simulink model "HystressisCurrentController"  (R2023a)
settings: Solver=VariableStepAuto  StartTime=0.0  StopTime=2  MaxStep=.001  RelTol=1e-3
values from neighbouring files (symbols this model uses):
  B = .005752    (= 0.005752)    [parameters.m]
  Delta = 0.1    [parameters.m]
  J = .02    (= 0.02)    [parameters.m]
  lambda_r_rated = (Vph_rms/(2*pi*Freq))*(1-sigma)    [parameters.m]
  Llr = .005974    (= 0.005974)    [parameters.m]
  Lls = .005974    (= 0.005974)    [parameters.m]
  Lm = .2037    (= 0.2037)    [parameters.m]
  Lr = Lm+Llr    (= 0.209674)    [parameters.m]
  P = 4    [parameters.m]
  Rs = 1.115    [parameters.m]
  Tr = Lr/Rr    (= 0.193604801477)    [parameters.m]
  Vdc = 400    [parameters.m]
libraries: spsMosfetLib x6, spsabctoAlphaBetaZeroLib x4, slpidlib x4, spsAsynchronousMachineSIUnitsLib x1, spsDCVoltageSourceLib x1, spsGroundLib x1, SignalEditorBlockLib x1, spsThreePhaseVIMeasurementLib x1, spsabctodq0Lib x1, sps_lib x1
settings Model: Creator=User  LastModifiedBy=User

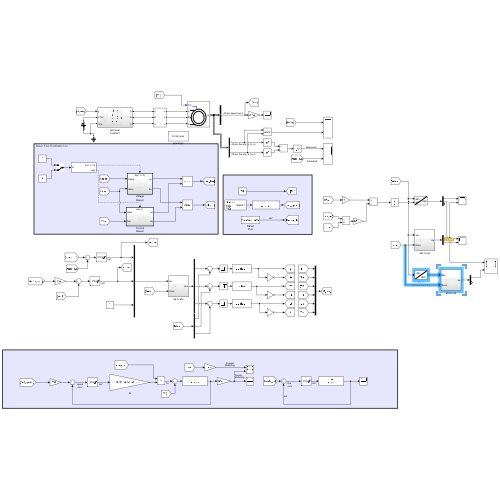
[thumbnail: Simulink's stored preview of the top-level diagram]
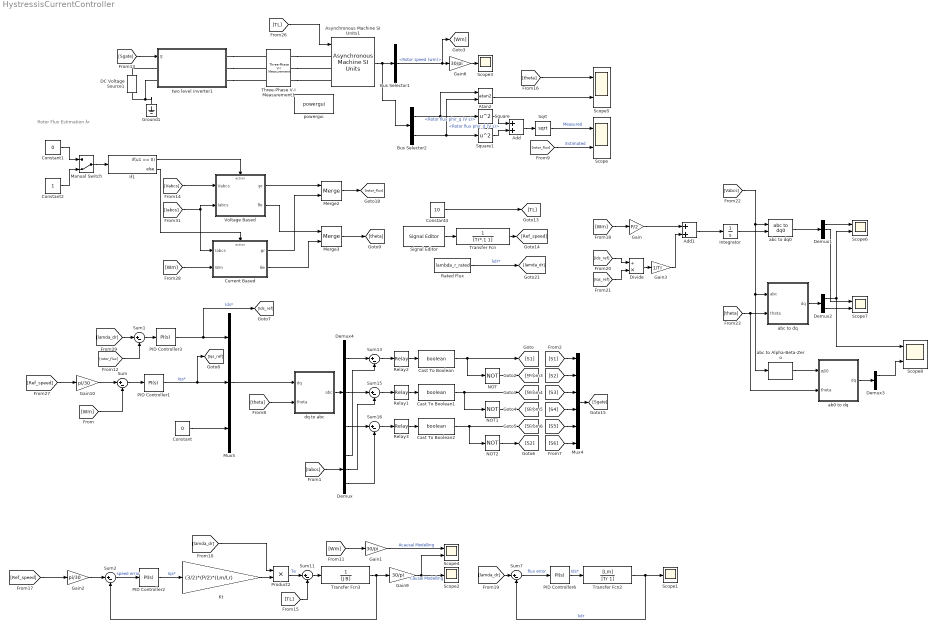
== system HystressisCurrentController ==
  note: Rotor Flux Estimation λr
  Add : Sum
  Add1 : Sum
  Asynchronous Machine SI Units1 : spsAsynchronousMachineSIUnitsLib/Asynchronous Machine SI Units  RotorType=Squirrel-cage  PresetModel="01:  5 HP   460 V 60Hz 1750 RPM"  MechanicalLoad=Torque Tm  ShowDetailedParameters=on  ReferenceFrame=Stationary  Units=SI  MeasurementBus=off  NominalParameters=[3730 460 60]  VoltageRatio=1  Stator=[1.115 0.005974]  Rotor=[1.083 0.005974]  Cage1=[0.4155 0.002066]  Cage2=[0.4168 0.0003495]  Lm=0.2037  Mechanical=[0.02 0.005752 2]  PolePairs=2  InitialConditions=[1 0 0 0 0 0 0 0]  SimulateSaturation=off  Saturation=[14.03593122, 27.81365428, 53.79336849, 72.68890987, 97.98006896, 148.6815601, 215.7428561, 302.9841135, 428.7778367 ; 230, 322, 414, 460, 506, 552, 598, 644, 690]  LoadFlowParameters=1492000  TsPowergui=0  TsBlock=-1  IterativeModel=Trapezoidal non iterative  IterativeDiscreteModel=Trapezoidal non iterative  Pmec=1.492e+006
  Atan2 : Trigonometry  Operator=atan2
  Bus Selector1 : BusSelector  OutputSignals=Mechanical.Rotor speed (wm)
  Bus Selector2 : BusSelector  OutputSignals=Rotor measurements.Rotor flux phir_q (V s),Rotor measurements.Rotor flux phir_d (V s)
  Cast To Boolean : DataTypeConversion  OutDataTypeStr=boolean  SaturateOnIntegerOverflow=off  RndMeth=Floor
  Cast To Boolean1 : DataTypeConversion  OutDataTypeStr=boolean  SaturateOnIntegerOverflow=off  RndMeth=Floor
  Cast To Boolean2 : DataTypeConversion  OutDataTypeStr=boolean  SaturateOnIntegerOverflow=off  RndMeth=Floor
  Constant : Constant  Value=0
  Constant1 : Constant  Value=0
  Constant2 : Constant
  Constant4 : Constant  Value=10
  Current Based : Subsystem
  DC Voltage Source1 : spsDCVoltageSourceLib/DC Voltage Source  Amplitude=Vdc  Measurements=None
  Demux : Demux  Outputs=3
  Demux1 : Demux  Outputs=3
  Demux2 : Demux  Outputs=2
  Demux3 : Demux  Outputs=2
  Demux4 : Demux  Outputs=3
  Divide : Product  Inputs=/*
  Gain : Gain  Gain=P/2
  Gain1 : Gain  Gain=30/pi
  Gain10 : Gain  Gain=pi/30
  Gain2 : Gain  Gain=pi/30
  Gain3 : Gain  Gain=1/Tr
  Gain6 : Gain  Gain=30/pi
  Gain9 : Gain  Gain=30/pi
  Ground1 : spsGroundLib/Ground  LConnTagsString=a
  If1 : If  IfExpression=u1 == 0
  Integrator : Integrator
  Kt : Gain  Gain=(3/2)*(P/2)*(Lm/Lr)
  Manual Switch : ManualSwitch  CurrentSetting=0
  Merge2 : Merge
  Merge3 : Merge
  Mux4 : Mux  Inputs=6
  Mux5 : Mux  Inputs=3
  NOT : Logic  Operator=NOT  IconShape=distinctive  AllPortsSameDT=off  OutDataTypeStr=boolean
  NOT1 : Logic  Operator=NOT  IconShape=distinctive  AllPortsSameDT=off  OutDataTypeStr=boolean
  NOT2 : Logic  Operator=NOT  IconShape=distinctive  AllPortsSameDT=off  OutDataTypeStr=boolean
  PID Controller1 : slpidlib/PID Controller  Controller=PI  Form=Parallel  TimeDomain=Continuous-time  UseExternalTs=off  SampleTime=-1  IntegratorMethod=Forward Euler  FilterMethod=Forward Euler  ControllerParametersSource=internal  P=5.28558902613874  I=47.3840704653277  UseKiTs=off  D=0  N=100  UseFilter=on  TunerSelectOption=Transfer Function Based (PID Tuner App)  InitialConditionSource=internal  InitialConditionForIntegrator=0  InitialConditionForFilter=0  DifferentiatorICPrevScaledInput=0  ExternalReset=none  TrackingMode=off  Kt=1  LimitOutput=on  SatLimitsSource=internal  UpperSaturationLimit=inf  LowerSaturationLimit=-inf  LinearizeAsGain=on  AntiWindupMode=clamping  Kb=1  LimitIntegrator=off  UpperIntegratorSaturationLimit=inf  LowerIntegratorSaturationLimit=-inf  POutMin=[]  POutMax=[]  IOutMin=[]  IOutMax=[]  DOutMin=[]  DOutMax=[]  NOutMin=[]  NOutMax=[]  SumOutMin=[]  SumOutMax=[]  SaturationOutMin=[]  SaturationOutMax=[]  PParamMin=[]  PParamMax=[]  IParamMin=[]  IParamMax=[]  DParamMin=[]  DParamMax=[]  NParamMin=[]  NParamMax=[]  KbParamMin=[]  KbParamMax=[]  KtParamMin=[]  KtParamMax=[]  KbOutMin=[]  KbOutMax=[]  KtOutMin=[]  KtOutMax=[]  IntegratorOutMin=[]  IntegratorOutMax=[]  FilterOutMin=[]  FilterOutMax=[]  SumI1OutMin=[]  SumI1OutMax=[]  SumI2OutMin=[]  SumI2OutMax=[]  SumI3OutMin=[]  SumI3OutMax=[]  SumI4OutMin=[]  SumI4OutMax=[]  SumDOutMin=[]  SumDOutMax=[]  DifferentiatorOutMin=[]  DifferentiatorOutMax=[]  FilterDiffOutCoefMin=[]  FilterDiffOutCoefMax=[]  ReciprocalOutMin=[]  ReciprocalOutMax=[]  SumDenOutMin=[]  SumDenOutMax=[]  SumNumOutMin=[]  SumNumOutMax=[]  DivideOutMin=[]  DivideOutMax=[]  UdiffTsProdOutMin=[]  UdiffTsProdOutMax=[]  NTsProdOutMin=[]  NTsProdOutMax=[]  UintegralTsProdOutMin=[]  UintegralTsProdOutMax=[]  UngainTsProdOutMin=[]  UngainTsProdOutMax=[]  ClampingZeroOutDataTypeStr=Inherit: Inherit via back propagation  ClampingZeroOutMin=[]  ClampingZeroOutMax=[]  FilterDenConstantOutDataTypeStr=Inherit: Inherit via back propagation  FilterDenConstantOutMin=[]  FilterDenConstantOutMax=[]  PCopyOutDataTypeStr=Inherit: Inherit via back propagation  PCopyOutMin=[]  PCopyOutMax=[]  NCopyOutDataTypeStr=Inherit: Inherit via back propagation  NCopyOutMin=[]  NCopyOutMax=[]  IntegratorContinuousStateAttributes=''  IntegratorStateMustResolveToSignalObject=off  IntegratorRTWStateStorageClass=Auto  FilterContinuousStateAttributes=''  FilterStateMustResolveToSignalObject=off  FilterRTWStateStorageClass=Auto  ParallelPVariant=InternalParameters  IdealPVariant=Disabled  IVariant=InternalParameters  DVariant=Disabled  IntegratorVariant=Continuous  SatVariant=Enabled  AWVariant=ContClampingParallel  PCopyVariant=Disabled  TRVariant=Disabled  FdbkBlocksVariant=Forward  IdealPFdbkVariant=Disabled  SatFdbkVariant=Disabled  DerivativeFilterVariant=Disabled  NVariant=Disabled  NCopyVariant=Disabled_SignalSpec  FilterICVariant=Disabled  IntegratorICVariant=InternalICs  ExternalResetVariant=Disabled  TRSumVariant=Passthrough  SumFdbkVariant=Disabled  SumVariant=Sum_PI  TsampFilterVariant=InternalTs  TsampNgainVariant=Passthrough  TsampIntegralVariant=Disabled_SignalSpec  ExternalSaturationOutDataTypeStr=Inherit: Same as second input
  PID Controller2 : slpidlib/PID Controller  Controller=PI  Form=Parallel  TimeDomain=Continuous-time  UseExternalTs=off  SampleTime=-1  IntegratorMethod=Forward Euler  FilterMethod=Forward Euler  ControllerParametersSource=internal  P=5.28558902613874  I=47.3840704653277  UseKiTs=off  D=0  N=100  UseFilter=on  TunerSelectOption=Transfer Function Based (PID Tuner App)  InitialConditionSource=internal  InitialConditionForIntegrator=0  InitialConditionForFilter=0  DifferentiatorICPrevScaledInput=0  ExternalReset=none  TrackingMode=off  Kt=1  LimitOutput=on  SatLimitsSource=internal  UpperSaturationLimit=inf  LowerSaturationLimit=-inf  LinearizeAsGain=on  AntiWindupMode=clamping  Kb=1  LimitIntegrator=off  UpperIntegratorSaturationLimit=inf  LowerIntegratorSaturationLimit=-inf  POutMin=[]  POutMax=[]  IOutMin=[]  IOutMax=[]  DOutMin=[]  DOutMax=[]  NOutMin=[]  NOutMax=[]  SumOutMin=[]  SumOutMax=[]  SaturationOutMin=[]  SaturationOutMax=[]  PParamMin=[]  PParamMax=[]  IParamMin=[]  IParamMax=[]  DParamMin=[]  DParamMax=[]  NParamMin=[]  NParamMax=[]  KbParamMin=[]  KbParamMax=[]  KtParamMin=[]  KtParamMax=[]  KbOutMin=[]  KbOutMax=[]  KtOutMin=[]  KtOutMax=[]  IntegratorOutMin=[]  IntegratorOutMax=[]  FilterOutMin=[]  FilterOutMax=[]  SumI1OutMin=[]  SumI1OutMax=[]  SumI2OutMin=[]  SumI2OutMax=[]  SumI3OutMin=[]  SumI3OutMax=[]  SumI4OutMin=[]  SumI4OutMax=[]  SumDOutMin=[]  SumDOutMax=[]  DifferentiatorOutMin=[]  DifferentiatorOutMax=[]  FilterDiffOutCoefMin=[]  FilterDiffOutCoefMax=[]  ReciprocalOutMin=[]  ReciprocalOutMax=[]  SumDenOutMin=[]  SumDenOutMax=[]  SumNumOutMin=[]  SumNumOutMax=[]  DivideOutMin=[]  DivideOutMax=[]  UdiffTsProdOutMin=[]  UdiffTsProdOutMax=[]  NTsProdOutMin=[]  NTsProdOutMax=[]  UintegralTsProdOutMin=[]  UintegralTsProdOutMax=[]  UngainTsProdOutMin=[]  UngainTsProdOutMax=[]  ClampingZeroOutDataTypeStr=Inherit: Inherit via back propagation  ClampingZeroOutMin=[]  ClampingZeroOutMax=[]  FilterDenConstantOutDataTypeStr=Inherit: Inherit via back propagation  FilterDenConstantOutMin=[]  FilterDenConstantOutMax=[]  PCopyOutDataTypeStr=Inherit: Inherit via back propagation  PCopyOutMin=[]  PCopyOutMax=[]  NCopyOutDataTypeStr=Inherit: Inherit via back propagation  NCopyOutMin=[]  NCopyOutMax=[]  IntegratorContinuousStateAttributes=''  IntegratorStateMustResolveToSignalObject=off  IntegratorRTWStateStorageClass=Auto  FilterContinuousStateAttributes=''  FilterStateMustResolveToSignalObject=off  FilterRTWStateStorageClass=Auto  ParallelPVariant=InternalParameters  IdealPVariant=Disabled  IVariant=InternalParameters  DVariant=Disabled  IntegratorVariant=Continuous  SatVariant=Enabled  AWVariant=ContClampingParallel  PCopyVariant=Disabled  TRVariant=Disabled  FdbkBlocksVariant=Forward  IdealPFdbkVariant=Disabled  SatFdbkVariant=Disabled  DerivativeFilterVariant=Disabled  NVariant=Disabled  NCopyVariant=Disabled_SignalSpec  FilterICVariant=Disabled  IntegratorICVariant=InternalICs  ExternalResetVariant=Disabled  TRSumVariant=Passthrough  SumFdbkVariant=Disabled  SumVariant=Sum_PI  TsampFilterVariant=InternalTs  TsampNgainVariant=Passthrough  TsampIntegralVariant=Disabled_SignalSpec  ExternalSaturationOutDataTypeStr=Inherit: Same as second input
  PID Controller3 : slpidlib/PID Controller  Controller=PI  Form=Parallel  TimeDomain=Continuous-time  UseExternalTs=off  SampleTime=-1  IntegratorMethod=Forward Euler  FilterMethod=Forward Euler  ControllerParametersSource=internal  P=247.450327990912  I=1324.30326231712  UseKiTs=off  D=0  N=100  UseFilter=on  TunerSelectOption=Transfer Function Based (PID Tuner App)  InitialConditionSource=internal  InitialConditionForIntegrator=0  InitialConditionForFilter=0  DifferentiatorICPrevScaledInput=0  ExternalReset=none  TrackingMode=off  Kt=1  LimitOutput=on  SatLimitsSource=internal  UpperSaturationLimit=inf  LowerSaturationLimit=-inf  LinearizeAsGain=on  AntiWindupMode=clamping  Kb=1  LimitIntegrator=off  UpperIntegratorSaturationLimit=inf  LowerIntegratorSaturationLimit=-inf  POutMin=[]  POutMax=[]  IOutMin=[]  IOutMax=[]  DOutMin=[]  DOutMax=[]  NOutMin=[]  NOutMax=[]  SumOutMin=[]  SumOutMax=[]  SaturationOutMin=[]  SaturationOutMax=[]  PParamMin=[]  PParamMax=[]  IParamMin=[]  IParamMax=[]  DParamMin=[]  DParamMax=[]  NParamMin=[]  NParamMax=[]  KbParamMin=[]  KbParamMax=[]  KtParamMin=[]  KtParamMax=[]  KbOutMin=[]  KbOutMax=[]  KtOutMin=[]  KtOutMax=[]  IntegratorOutMin=[]  IntegratorOutMax=[]  FilterOutMin=[]  FilterOutMax=[]  SumI1OutMin=[]  SumI1OutMax=[]  SumI2OutMin=[]  SumI2OutMax=[]  SumI3OutMin=[]  SumI3OutMax=[]  SumI4OutMin=[]  SumI4OutMax=[]  SumDOutMin=[]  SumDOutMax=[]  DifferentiatorOutMin=[]  DifferentiatorOutMax=[]  FilterDiffOutCoefMin=[]  FilterDiffOutCoefMax=[]  ReciprocalOutMin=[]  ReciprocalOutMax=[]  SumDenOutMin=[]  SumDenOutMax=[]  SumNumOutMin=[]  SumNumOutMax=[]  DivideOutMin=[]  DivideOutMax=[]  UdiffTsProdOutMin=[]  UdiffTsProdOutMax=[]  NTsProdOutMin=[]  NTsProdOutMax=[]  UintegralTsProdOutMin=[]  UintegralTsProdOutMax=[]  UngainTsProdOutMin=[]  UngainTsProdOutMax=[]  ClampingZeroOutDataTypeStr=Inherit: Inherit via back propagation  ClampingZeroOutMin=[]  ClampingZeroOutMax=[]  FilterDenConstantOutDataTypeStr=Inherit: Inherit via back propagation  FilterDenConstantOutMin=[]  FilterDenConstantOutMax=[]  PCopyOutDataTypeStr=Inherit: Inherit via back propagation  PCopyOutMin=[]  PCopyOutMax=[]  NCopyOutDataTypeStr=Inherit: Inherit via back propagation  NCopyOutMin=[]  NCopyOutMax=[]  IntegratorContinuousStateAttributes=''  IntegratorStateMustResolveToSignalObject=off  IntegratorRTWStateStorageClass=Auto  FilterContinuousStateAttributes=''  FilterStateMustResolveToSignalObject=off  FilterRTWStateStorageClass=Auto  ParallelPVariant=InternalParameters  IdealPVariant=Disabled  IVariant=InternalParameters  DVariant=Disabled  IntegratorVariant=Continuous  SatVariant=Enabled  AWVariant=ContClampingParallel  PCopyVariant=Disabled  TRVariant=Disabled  FdbkBlocksVariant=Forward  IdealPFdbkVariant=Disabled  SatFdbkVariant=Disabled  DerivativeFilterVariant=Disabled  NVariant=Disabled  NCopyVariant=Disabled_SignalSpec  FilterICVariant=Disabled  IntegratorICVariant=InternalICs  ExternalResetVariant=Disabled  TRSumVariant=Passthrough  SumFdbkVariant=Disabled  SumVariant=Sum_PI  TsampFilterVariant=InternalTs  TsampNgainVariant=Passthrough  TsampIntegralVariant=Disabled_SignalSpec  ExternalSaturationOutDataTypeStr=Inherit: Same as second input
  PID Controller6 : slpidlib/PID Controller  Controller=PI  Form=Parallel  TimeDomain=Continuous-time  UseExternalTs=off  SampleTime=-1  IntegratorMethod=Forward Euler  FilterMethod=Forward Euler  ControllerParametersSource=internal  P=247.450327990912  I=1324.30326231712  UseKiTs=off  D=0  N=100  UseFilter=on  TunerSelectOption=Transfer Function Based (PID Tuner App)  InitialConditionSource=internal  InitialConditionForIntegrator=0  InitialConditionForFilter=0  DifferentiatorICPrevScaledInput=0  ExternalReset=none  TrackingMode=off  Kt=1  LimitOutput=on  SatLimitsSource=internal  UpperSaturationLimit=inf  LowerSaturationLimit=-inf  LinearizeAsGain=on  AntiWindupMode=clamping  Kb=1  LimitIntegrator=off  UpperIntegratorSaturationLimit=inf  LowerIntegratorSaturationLimit=-inf  POutMin=[]  POutMax=[]  IOutMin=[]  IOutMax=[]  DOutMin=[]  DOutMax=[]  NOutMin=[]  NOutMax=[]  SumOutMin=[]  SumOutMax=[]  SaturationOutMin=[]  SaturationOutMax=[]  PParamMin=[]  PParamMax=[]  IParamMin=[]  IParamMax=[]  DParamMin=[]  DParamMax=[]  NParamMin=[]  NParamMax=[]  KbParamMin=[]  KbParamMax=[]  KtParamMin=[]  KtParamMax=[]  KbOutMin=[]  KbOutMax=[]  KtOutMin=[]  KtOutMax=[]  IntegratorOutMin=[]  IntegratorOutMax=[]  FilterOutMin=[]  FilterOutMax=[]  SumI1OutMin=[]  SumI1OutMax=[]  SumI2OutMin=[]  SumI2OutMax=[]  SumI3OutMin=[]  SumI3OutMax=[]  SumI4OutMin=[]  SumI4OutMax=[]  SumDOutMin=[]  SumDOutMax=[]  DifferentiatorOutMin=[]  DifferentiatorOutMax=[]  FilterDiffOutCoefMin=[]  FilterDiffOutCoefMax=[]  ReciprocalOutMin=[]  ReciprocalOutMax=[]  SumDenOutMin=[]  SumDenOutMax=[]  SumNumOutMin=[]  SumNumOutMax=[]  DivideOutMin=[]  DivideOutMax=[]  UdiffTsProdOutMin=[]  UdiffTsProdOutMax=[]  NTsProdOutMin=[]  NTsProdOutMax=[]  UintegralTsProdOutMin=[]  UintegralTsProdOutMax=[]  UngainTsProdOutMin=[]  UngainTsProdOutMax=[]  ClampingZeroOutDataTypeStr=Inherit: Inherit via back propagation  ClampingZeroOutMin=[]  ClampingZeroOutMax=[]  FilterDenConstantOutDataTypeStr=Inherit: Inherit via back propagation  FilterDenConstantOutMin=[]  FilterDenConstantOutMax=[]  PCopyOutDataTypeStr=Inherit: Inherit via back propagation  PCopyOutMin=[]  PCopyOutMax=[]  NCopyOutDataTypeStr=Inherit: Inherit via back propagation  NCopyOutMin=[]  NCopyOutMax=[]  IntegratorContinuousStateAttributes=''  IntegratorStateMustResolveToSignalObject=off  IntegratorRTWStateStorageClass=Auto  FilterContinuousStateAttributes=''  FilterStateMustResolveToSignalObject=off  FilterRTWStateStorageClass=Auto  ParallelPVariant=InternalParameters  IdealPVariant=Disabled  IVariant=InternalParameters  DVariant=Disabled  IntegratorVariant=Continuous  SatVariant=Enabled  AWVariant=ContClampingParallel  PCopyVariant=Disabled  TRVariant=Disabled  FdbkBlocksVariant=Forward  IdealPFdbkVariant=Disabled  SatFdbkVariant=Disabled  DerivativeFilterVariant=Disabled  NVariant=Disabled  NCopyVariant=Disabled_SignalSpec  FilterICVariant=Disabled  IntegratorICVariant=InternalICs  ExternalResetVariant=Disabled  TRSumVariant=Passthrough  SumFdbkVariant=Disabled  SumVariant=Sum_PI  TsampFilterVariant=InternalTs  TsampNgainVariant=Passthrough  TsampIntegralVariant=Disabled_SignalSpec  ExternalSaturationOutDataTypeStr=Inherit: Same as second input
  Product2 : Product
  Rated Flux : Constant  Value=lambda_r_rated
  Relay1 : Relay  OnSwitchValue=Delta/2  OffSwitchValue=(-1*Delta)/2
  Relay2 : Relay  OnSwitchValue=Delta/2  OffSwitchValue=(-1*Delta)/2
  Relay3 : Relay  OnSwitchValue=Delta/2  OffSwitchValue=(-1*Delta)/2
  Scope{,4..8} (6 alike) : Scope  NumInputPorts=2
  Scope1 : Scope
  Scope2 : Scope
  Scope3 : Scope
  Signal Editor : SignalEditorBlockLib/Signal Editor  FileName=speedRef.mat  ActiveScenario=Scenario  ActiveSignal=Signal 1  IsBus=off  OutputBusObjectStr=Bus: BusObject  SampleTime=0  Interpolate=off  ZeroCross=off  OutputAfterFinalValue=Setting to zero  Unit=inherit  PreserveSignalName=on  ApplySigPropsToAllScenarios=on
  Sqrt : Sqrt
  Square : Math  Operator=square
  Square1 : Math  Operator=square
  Sum{,1..2,7,11,13,15..16} (8 alike) : Sum  Inputs=|+-
  Three-Phase V-I Measurement1 : spsThreePhaseVIMeasurementLib/Three-Phase V-I Measurement  VoltageMeasurement=phase-to-ground  SetLabelV=on  LabelV=Vabcs  Vpu=off  VpuLL=off  CurrentMeasurement=yes  SetLabelI=on  LabelI=Iabcs  Ipu=off  Pbase=100e6  Vbase=500e3  OutputType=Complex  PhasorSimulation=off  PSBequivalent=0
  Transfer Fcn : TransferFcn  Denominator=[Tr*.1 1]
  Transfer Fcn2 : TransferFcn  Numerator=[Lm]  Denominator=[Tr 1]
  Transfer Fcn3 : TransferFcn  Denominator=[J B]
  Voltage Based : Subsystem
  ab0 to dq : Subsystem
  abc to Alpha-Beta-Zero : spsabctoAlphaBetaZeroLib/abc to Alpha-Beta-Zero
  abc to dq : Subsystem
  abc to dq0 : spsabctodq0Lib/abc to dq0  Alignment=Aligned with phase A axis
  dq to abc : Subsystem
  powergui : sps_lib/powergui  Priority=1  SimulationMode=Continuous  SampleTime=50e-6  frequency=60  Iterations=50  frequencyindice=60  Pbase=100e6  ErrMax=1e-4  UnitsV=kV  UnitsW=MW  buscounter=0  FunctionMessages=off  echomessages=off  EnableUseOfTLC=off  CurrentSourceSwitches=off  DisableSnubberDevices=off  DisableRonSwitches=off  DisableVfSwitches=off  DisplayEquations=off  AutomaticDiscreteSolvers=off  SolverType=Tustin/Backward Euler (TBE)  Interpol=off  ExternalGateDelay=off  methode=off  Ts=100  x0status=blocks  SPID=on  SwTol=0  HookPort=off  NonlinearTolerance=1e-4  nMaxIteration=100  ContinueOnMaxIteration=off  RestoreLinks=warning  ResistiveCurrentMeasurement=off  Frange=[0:2:500]  Ylog=off  Xlog=on  ShowGrid=off  save=off  variable=ZData  structure=0  ZoomFFT=off  StartTime=0.0  cycles=1  DisplayStyle=1  fundamental=60  FreqAxis=off  MaxFrequency=1000  frequencyindicesteady=1  RmsSteady=1  display=off
  two level inverter1 : Subsystem
  wires:
  Mux4/1 -> [Sgate]
  Demux4/2 -> Sum15/1
  dq to abc/1(abc) -> Demux4/1
  Sum16/1 -> Relay3/1
  Relay1/1 -> Cast To Boolean1/1
  Sum1/1 -> PID Controller3/1
  Sum15/1 -> Relay1/1
  Constant/1 -> Mux5/3
  [TL] -> Asynchronous Machine SI Units1/1
  Gain10/1 -> Sum/1
  Current Based/1(φr) -> Merge2/2
  Merge3/1 -> [theta]
  Current Based/2(θe) -> Merge3/2
  Bus Selector1/1 -> Gain6/1, [Wm]  "<Rotor speed (wm)>"
  Constant4/1 -> [TL]
  Gain6/1 -> Scope3/1
  Asynchronous Machine SI Units1/1 -> Bus Selector2/1, Bus Selector1/1
  [Wm] -> Current Based/2(Wm)
  Voltage Based/2(θe) -> Merge3/1
  Rated Flux/1 -> [lamda_dr]  "λdr*"
  If1/1 -> Voltage Based/Action
  Voltage Based/1(φr) -> Merge2/1
  Sum/1 -> PID Controller1/1
  [Vabcs] -> Voltage Based/1(Vabcs)
  Relay3/1 -> Cast To Boolean2/1
  Merge2/1 -> [rotor_flux]
  [Ref_speed] -> Gain10/1
  Demux4/3 -> Sum16/1
  Demux4/1 -> Sum13/1
  [Iabcs] -> Voltage Based/2(Iabcs), Current Based/1(Iabcs)
  Relay2/1 -> Cast To Boolean/1
  [Sgate] -> two level inverter1/1(g)
  PID Controller1/1 -> [Iqs_ref], Mux5/2  "Iqs*"
  If1/2 -> Current Based/Action
  [Wm] -> Sum/2
  NOT/1 -> [S4]
  NOT1/1 -> [S6]
  NOT2/1 -> [S2]
  [Iabcs] -> Demux/1
  Demux/1 -> Sum13/2
  Demux/2 -> Sum15/2
  Demux/3 -> Sum16/2
  [S1] -> Mux4/1
  [S2] -> Mux4/2
  [S3] -> Mux4/3
  [S4] -> Mux4/4
  [S5] -> Mux4/5
  [S6] -> Mux4/6
  Cast To Boolean/1 -> [S1], NOT/1
  Cast To Boolean1/1 -> [S3], NOT1/1
  Cast To Boolean2/1 -> NOT2/1, [S5]
  Sum13/1 -> Relay2/1
  Mux5/1 -> dq to abc/1(dq)
  [lamda_dr] -> Sum1/1
  [theta] -> dq to abc/2(theta)
  Bus Selector2/1 -> Atan2/1, Square/1  "<Rotor flux phir_q (V s)>"
  Bus Selector2/2 -> Atan2/2, Square1/1  "<Rotor flux phir_d (V s)>"
  Square/1 -> Add/1
  Square1/1 -> Add/2
  Add/1 -> Sqrt/1
  Sqrt/1 -> Scope/1  "Measured"
  [rotor_flux] -> Scope/2  "Estimated"
  Transfer Fcn3/1 -> Gain9/1, Sum2/2
  [TL] -> Sum11/2
  Kt/1 -> Product2/2
  Sum11/1 -> Transfer Fcn3/1
  Transfer Fcn2/1 -> Scope1/1, Sum7/2  "λdr"
  Sum7/1 -> PID Controller6/1  "flux error"
  Gain2/1 -> Sum2/1
  Product2/1 -> Sum11/1  "Te"
  Gain9/1 -> Scope4/2, Scope2/1  "Causal Modelling"
  Sum2/1 -> PID Controller2/1  "speed error"
  PID Controller2/1 -> Kt/1  "Iqs*"
  [lamda_dr] -> Product2/1
  [lamda_dr] -> Sum7/1
  [Ref_speed] -> Gain2/1
  PID Controller6/1 -> Transfer Fcn2/1  "Ids*"
  [Wm] -> Gain1/1
  Gain1/1 -> Scope4/1  "Acausal Modelling"
  PID Controller3/1 -> [Ids_ref], Mux5/1  "Ids*"
  [rotor_flux] -> Sum1/2
  Transfer Fcn/1 -> [Ref_speed]
  Atan2/1 -> Scope5/2
  [theta] -> Scope5/1
  Signal Editor/1 -> Transfer Fcn/1
  Manual Switch/1 -> If1/1
  Constant1/1 -> Manual Switch/1
  Constant2/1 -> Manual Switch/2
  [Wm] -> Gain/1
  Gain/1 -> Add1/1
  [Ids_ref] -> Divide/1
  [Iqs_ref] -> Divide/2
  Divide/1 -> Gain3/1
  Gain3/1 -> Add1/2
  Add1/1 -> Integrator/1
  [Vabcs] -> abc to Alpha-Beta-Zero/1, abc to dq/1(abc), abc to dq0/1
  abc to dq0/1 -> Demux1/1
  [theta] -> ab0 to dq/2(theta), abc to dq/2(theta)
  abc to dq/1(dq) -> Demux2/1
  Demux2/2 -> Scope7/2
  Demux1/2 -> Scope7/1
  Integrator/1 -> abc to dq0/2
  abc to Alpha-Beta-Zero/1 -> ab0 to dq/1(αβ0)
  ab0 to dq/1(dq) -> Demux3/1
  Demux3/1 -> Scope8/2
  Demux1/1 -> Scope6/1
  Demux2/1 -> Scope6/2, Scope8/1
  connections:
  Ground1/LConn1 -- two level inverter1/LConn2 -- DC Voltage Source1/LConn1
  Three-Phase V-I Measurement1/RConn2 -- Asynchronous Machine SI Units1/LConn2
  two level inverter1/RConn3 -- Three-Phase V-I Measurement1/LConn3
  Three-Phase V-I Measurement1/RConn3 -- Asynchronous Machine SI Units1/LConn3
  Three-Phase V-I Measurement1/RConn1 -- Asynchronous Machine SI Units1/LConn1
  two level inverter1/RConn2 -- Three-Phase V-I Measurement1/LConn2
  two level inverter1/RConn1 -- Three-Phase V-I Measurement1/LConn1
  DC Voltage Source1/RConn1 -- two level inverter1/LConn1

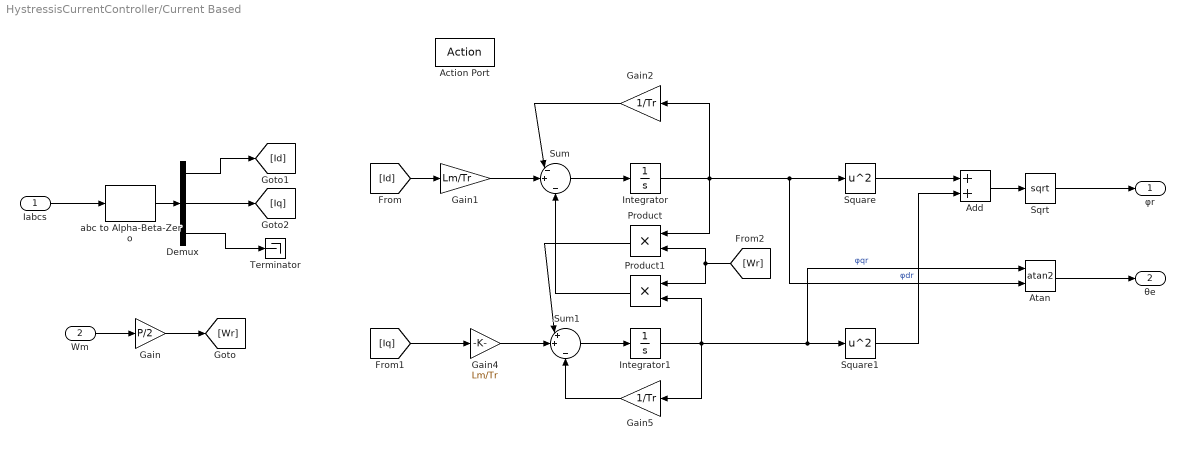
== system HystressisCurrentController/Current Based ==
  Iabcs : Inport
  Wm : Inport  Port=2
  Action Port : ActionPort  ActionPortLabel=else
  Add : Sum
  Atan : Trigonometry  Operator=atan2
  Demux : Demux  Outputs=3
  Gain : Gain  Gain=P/2
  Gain1 : Gain  Gain=Lm/Tr
  Gain2 : Gain  Gain=1/Tr
  Gain4 : Gain  Gain=Lm/Tr
  Gain5 : Gain  Gain=1/Tr
  Integrator : Integrator
  Integrator1 : Integrator
  Product : Product
  Product1 : Product
  Sqrt : Sqrt
  Square : Math  Operator=square
  Square1 : Math  Operator=square
  Sum : Sum  Inputs=|-+|-
  Sum1 : Sum  Inputs=|++|-
  Terminator : Terminator
  abc to Alpha-Beta-Zero : spsabctoAlphaBetaZeroLib/abc to Alpha-Beta-Zero
  φr : Outport
  θe : Outport  Port=2
  wires:
  Atan/1 -> θe/1
  Sqrt/1 -> φr/1
  Add/1 -> Sqrt/1
  Square1/1 -> Add/2
  Square/1 -> Add/1
  Gain5/1 -> Sum1/3
  Integrator/1 -> Product/1, Gain2/1, Atan/2, Square/1  "φdr"
  Product/1 -> Sum1/1
  Product1/1 -> Sum/3
  Integrator1/1 -> Product1/2, Atan/1, Square1/1, Gain5/1  "φqr"
  [Wr] -> Product1/1, Product/2
  [Iq] -> Gain4/1
  Gain4/1 -> Sum1/2
  Sum1/1 -> Integrator1/1
  Gain2/1 -> Sum/1
  Sum/1 -> Integrator/1
  Gain1/1 -> Sum/2
  [Id] -> Gain1/1
  Demux/3 -> Terminator/1
  Demux/2 -> [Iq]
  Demux/1 -> [Id]
  abc to Alpha-Beta-Zero/1 -> Demux/1
  Iabcs/1 -> abc to Alpha-Beta-Zero/1
  Gain/1 -> [Wr]
  Wm/1 -> Gain/1

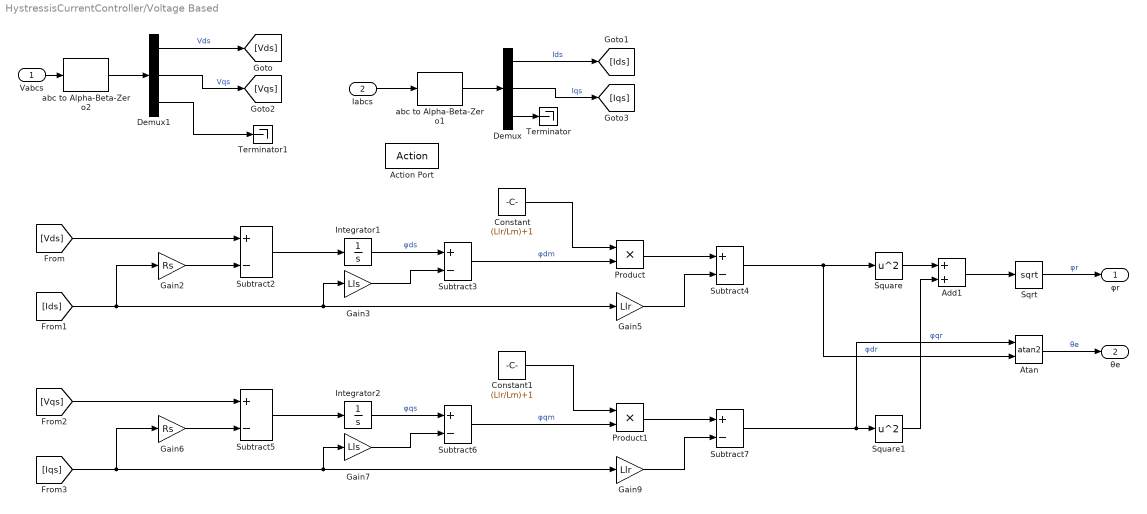
== system HystressisCurrentController/Voltage Based ==
  Vabcs : Inport
  Iabcs : Inport  Port=2
  Action Port : ActionPort  ActionPortLabel=if(u1 == 0)
  Add1 : Sum
  Atan : Trigonometry  Operator=atan2
  Constant : Constant  Value=(Llr/Lm)+1
  Constant1 : Constant  Value=(Llr/Lm)+1
  Demux : Demux  Outputs=3
  Demux1 : Demux  Outputs=3
  Gain2 : Gain  Gain=Rs
  Gain3 : Gain  Gain=Lls
  Gain5 : Gain  Gain=Llr
  Gain6 : Gain  Gain=Rs
  Gain7 : Gain  Gain=Lls
  Gain9 : Gain  Gain=Llr
  Integrator1 : Integrator
  Integrator2 : Integrator
  Product : Product
  Product1 : Product
  Sqrt : Sqrt
  Square : Math  Operator=square
  Square1 : Math  Operator=square
  Subtract{2..7} (6 alike) : Sum  Inputs=+-
  Terminator : Terminator
  Terminator1 : Terminator
  abc to Alpha-Beta-Zero1 : spsabctoAlphaBetaZeroLib/abc to Alpha-Beta-Zero
  abc to Alpha-Beta-Zero2 : spsabctoAlphaBetaZeroLib/abc to Alpha-Beta-Zero
  φr : Outport
  θe : Outport  Port=2
  wires:
  Iabcs/1 -> abc to Alpha-Beta-Zero1/1
  abc to Alpha-Beta-Zero1/1 -> Demux/1
  Demux/1 -> [Ids]  "Ids"
  Demux/2 -> [Iqs]  "Iqs"
  Demux1/2 -> [Vqs]  "Vqs"
  Demux1/1 -> [Vds]  "Vds"
  Demux/3 -> Terminator/1
  [Vds] -> Subtract2/1
  Gain2/1 -> Subtract2/2
  [Ids] -> Gain3/1, Gain5/1, Gain2/1
  Subtract2/1 -> Integrator1/1
  Integrator1/1 -> Subtract3/1  "φds"
  Gain3/1 -> Subtract3/2
  Subtract3/1 -> Product/2  "φdm"
  Constant/1 -> Product/1
  Product/1 -> Subtract4/1
  Gain5/1 -> Subtract4/2
  Subtract4/1 -> Atan/2, Square/1  "φdr"
  Subtract7/1 -> Atan/1, Square1/1  "φqr"
  Gain9/1 -> Subtract7/2
  Product1/1 -> Subtract7/1
  Subtract6/1 -> Product1/2  "φqm"
  Gain7/1 -> Subtract6/2
  Integrator2/1 -> Subtract6/1  "φqs"
  Subtract5/1 -> Integrator2/1
  [Iqs] -> Gain6/1, Gain9/1, Gain7/1
  Gain6/1 -> Subtract5/2
  [Vqs] -> Subtract5/1
  Square/1 -> Add1/1
  Add1/1 -> Sqrt/1
  Square1/1 -> Add1/2
  Sqrt/1 -> φr/1  "φr"
  Atan/1 -> θe/1  "θe"
  Constant1/1 -> Product1/1
  Vabcs/1 -> abc to Alpha-Beta-Zero2/1
  Demux1/3 -> Terminator1/1
  abc to Alpha-Beta-Zero2/1 -> Demux1/1

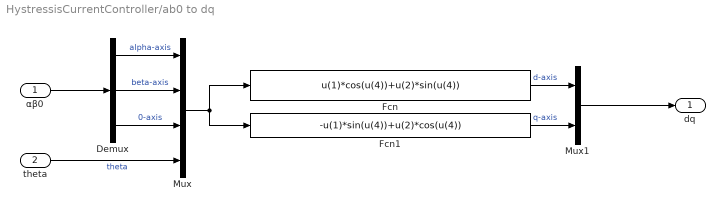
== system HystressisCurrentController/ab0 to dq ==
  αβ0 : Inport
  theta : Inport  Port=2
  Demux : Demux  Outputs=3
  Fcn : Fcn  Expr=u(1)*cos(u(4))+u(2)*sin(u(4))
  Fcn1 : Fcn  Expr=-u(1)*sin(u(4))+u(2)*cos(u(4))
  Mux : Mux
  Mux1 : Mux  Inputs=2
  dq : Outport
  wires:
  Mux/1 -> Fcn/1, Fcn1/1
  Fcn/1 -> Mux1/1  "d-axis"
  αβ0/1 -> Demux/1
  Demux/1 -> Mux/1  "alpha-axis"
  Demux/3 -> Mux/3  "0-axis"
  Demux/2 -> Mux/2  "beta-axis"
  theta/1 -> Mux/4  "theta"
  Fcn1/1 -> Mux1/2  "q-axis"
  Mux1/1 -> dq/1

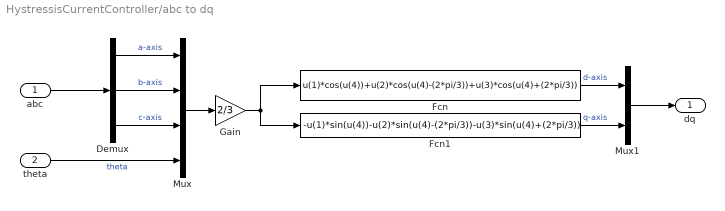
== system HystressisCurrentController/abc to dq ==
  abc : Inport
  theta : Inport  Port=2
  Demux : Demux  Outputs=3
  Fcn : Fcn  Expr=u(1)*cos(u(4))+u(2)*cos(u(4)-(2*pi/3))+u(3)*cos(u(4)+(2*pi/3))
  Fcn1 : Fcn  Expr=-u(1)*sin(u(4))-u(2)*sin(u(4)-(2*pi/3))-u(3)*sin(u(4)+(2*pi/3))
  Gain : Gain  Gain=2/3
  Mux : Mux
  Mux1 : Mux  Inputs=2
  dq : Outport
  wires:
  Mux1/1 -> dq/1
  Fcn1/1 -> Mux1/2  "q-axis"
  Mux/1 -> Gain/1
  theta/1 -> Mux/4  "theta"
  Demux/2 -> Mux/2  "b-axis"
  Demux/3 -> Mux/3  "c-axis"
  Demux/1 -> Mux/1  "a-axis"
  abc/1 -> Demux/1
  Fcn/1 -> Mux1/1  "d-axis"
  Gain/1 -> Fcn/1, Fcn1/1

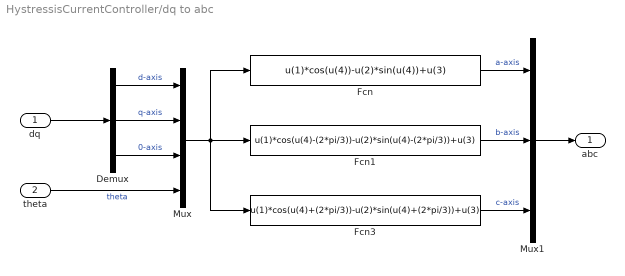
== system HystressisCurrentController/dq to abc ==
  dq : Inport
  theta : Inport  Port=2
  Demux : Demux  Outputs=3
  Fcn : Fcn  Expr=u(1)*cos(u(4))-u(2)*sin(u(4))+u(3)
  Fcn1 : Fcn  Expr=u(1)*cos(u(4)-(2*pi/3))-u(2)*sin(u(4)-(2*pi/3))+u(3)
  Fcn3 : Fcn  Expr=u(1)*cos(u(4)+(2*pi/3))-u(2)*sin(u(4)+(2*pi/3))+u(3)
  Mux : Mux
  Mux1 : Mux  Inputs=3
  abc : Outport
  wires:
  Fcn/1 -> Mux1/1  "a-axis"
  Fcn3/1 -> Mux1/3  "c-axis"
  dq/1 -> Demux/1
  Demux/1 -> Mux/1  "d-axis"
  Demux/3 -> Mux/3  "0-axis"
  Demux/2 -> Mux/2  "q-axis"
  theta/1 -> Mux/4  "theta"
  Mux/1 -> Fcn3/1, Fcn1/1, Fcn/1
  Fcn1/1 -> Mux1/2  "b-axis"
  Mux1/1 -> abc/1

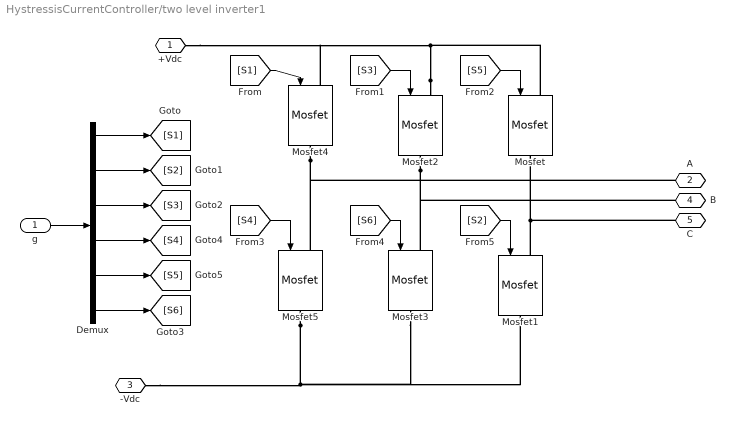
== system HystressisCurrentController/two level inverter1 ==
  g : Inport
  Demux : Demux  Outputs=6
  Mosfet{,1..5} (6 alike) : spsMosfetLib/Mosfet  Ron=0.1  Lon=0  Rd=0.01  Vfd=0  IC=0  Rs=1e5  Cs=inf  Measurements=off
  +Vdc : PMIOPort  Side=Left
  A : PMIOPort  Port=2  Side=Right
  -Vdc : PMIOPort  Port=3  Side=Left
  B : PMIOPort  Port=4  Side=Right
  C : PMIOPort  Port=5  Side=Right
  wires:
  [S2] -> Mosfet1/1
  [S6] -> Mosfet3/1
  [S4] -> Mosfet5/1
  [S5] -> Mosfet/1
  [S3] -> Mosfet2/1
  [S1] -> Mosfet4/1
  Demux/6 -> [S6]
  Demux/5 -> [S5]
  Demux/4 -> [S4]
  Demux/3 -> [S3]
  Demux/2 -> [S2]
  Demux/1 -> [S1]
  g/1 -> Demux/1
  connections:
  Mosfet4/RConn1 -- Mosfet5/LConn1 -- A/RConn1
  Mosfet2/RConn1 -- B/RConn1 -- Mosfet3/LConn1
  C/RConn1 -- Mosfet/RConn1 -- Mosfet1/LConn1
  Mosfet5/RConn1 -- -Vdc/RConn1 -- Mosfet1/RConn1 -- Mosfet3/RConn1
  Mosfet2/LConn1 -- Mosfet/LConn1 -- +Vdc/RConn1 -- Mosfet4/LConn1
